simulink library "Driveline_Axle2_A1_A2_A1Diff_A2Diff"  (R2025a)
settings: Solver=VariableStepAuto  StartTime=0.0  StopTime=10.0  RelTol=1e-3
undefined symbols (not defined in the file): ShaftA1, ShaftA2
libraries: Driveshaft_Assembly x4, Differential_Systems x2, fl_lib x2, sdl_lib x2
Description:
  | Component of Simscape Vehicle Templates Library
  | 
  | Copyright 2018-2025 The MathWorks, Inc.
settings Model: Creator=smiller  LastModifiedBy=smiller
settings SolverCC: AlgebraicLoopSolver=TrustRegion
settings DataIOCC: ReturnWorkspaceOutputs=off
settings OptimizationCC: ReuseModelBlockBuffer=off
settings DebuggingCC: UnconnectedInputMsg=warning  UnconnectedOutputMsg=warning  UnconnectedLineMsg=warning  ArithmeticOperatorsInVariantConditions=warning
settings ModelReferenceCC: EnableRefExpFcnMdlSchedulingChecks=on
settings SFSimCC: CustomCodeUndefinedFunction=UseInterfaceOnly
settings RTWCC: GPUComputeCapability=3.5  DLArmComputeVersion=19.05

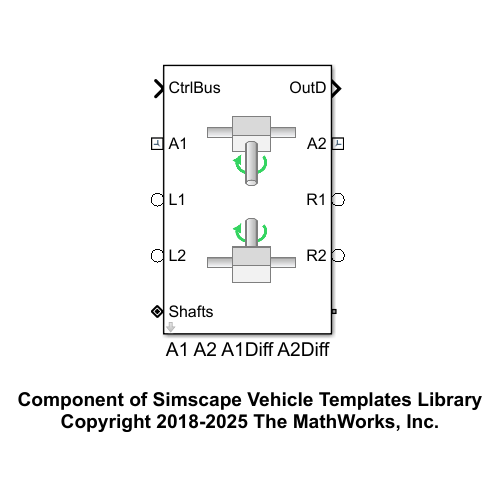
[thumbnail: Simulink's stored preview of the top-level diagram]
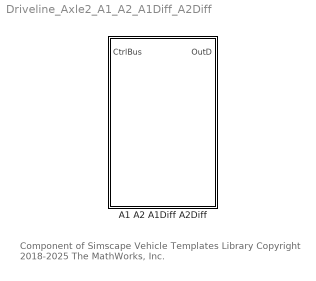
== system Driveline_Axle2_A1_A2_A1Diff_A2Diff ==
  note: Component of Simscape Vehicle Templates Library
      | Copyright 2018-2025 The MathWorks, Inc.
  A1 A2 A1Diff A2Diff : Subsystem  Tag=PublishSubsystem  VariantControl=IndepFRDiffFDiffR  mask(Driveline, Two-Axle, Two Input Shaft){}
      mask help: Models two-axle drivelines with differentials on front and rear axles.
      mask Display: image('sm_car_vehicle_driveline_axle2_a1_a2_a1diff_a2diff_IMAGE.png');

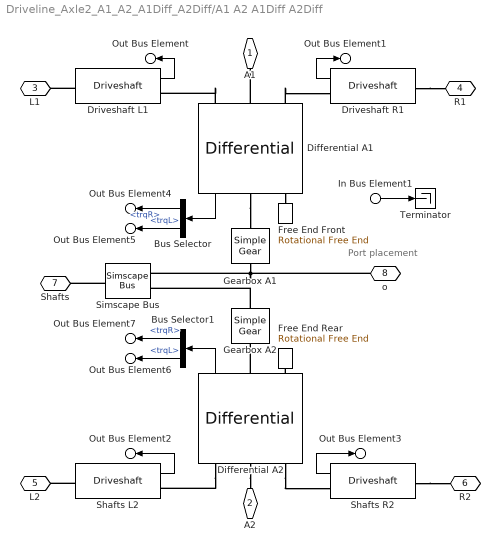
== system Driveline_Axle2_A1_A2_A1Diff_A2Diff/A1 A2 A1Diff A2Diff ==
  note: Port
      | placement
  In Bus Element1 : Inport  PortName=CtrlBus
  Bus Selector : BusSelector  OutputSignals=trqR,trqL
  Bus Selector1 : BusSelector  OutputSignals=trqR,trqL
  Differential A1 : Differential_Systems/Differential  VariantControl=Variant1  LabelModeActiveChoice=Gear1DShafts1D  Differential=Driveline.DifferentialA1  VariantLabel=Driveline.DifferentialA1.class.Value
      settings: AttributesFormatString=%<ActiveVariant>
  Differential A2 : Differential_Systems/Differential  VariantControl=Variant1  LabelModeActiveChoice=Gear1DShafts1D  Differential=Driveline.DifferentialA2  VariantLabel=Driveline.DifferentialA2.class.Value
      settings: AttributesFormatString=%<ActiveVariant>
  Driveshaft L1 : Driveshaft_Assembly/Driveshaft  VariantControl=Variant1  LabelModeActiveChoice=Shaft1D  popup_leftRight=Left  Driveshaft=Driveline.DriveshaftL1  VariantLabel=Driveline.DriveshaftL1.class.Value
      settings: AttributesFormatString=%<ActiveVariant>
  Driveshaft R1 : Driveshaft_Assembly/Driveshaft  VariantControl=Variant1  LabelModeActiveChoice=Shaft1D  popup_leftRight=Right  Driveshaft=Driveline.DriveshaftR1  VariantLabel=Driveline.DriveshaftR1.class.Value
      settings: AttributesFormatString=%<ActiveVariant>
  Free End Front : fl_lib/Mechanical/Rotational Elements/Rotational Free End  w_specify=off  w_priority=None  w=0 rad/s  w_nominal_specify=off  w_nominal_value=1  w_nominal_unit=rad/s
  Free End Rear : fl_lib/Mechanical/Rotational Elements/Rotational Free End  w_specify=off  w_priority=None  w=0 rad/s  w_nominal_specify=off  w_nominal_value=1  w_nominal_unit=rad/s
  Gearbox A1 : sdl_lib/Gears/Simple Gear  ratio=Driveline.GearboxA1.ratio.Value  rotation_direction=3-2*(1)  friction_model=1  T_noload=0.1 N*m  T_nom=5 N*m  efficiency_nom=0.8  efficiency=0.8  temperature_TLU=[280, 300, 320] K  load_TLU=[1, 5, 10] N*m  efficiency_TLU=[.95, .9, .85]  efficiency_TLU2=[.85, .8, .75; .95, .9, .85; .85, .8, .7]  w_thr=0.01 rad/s  pwr_thr=0.001 W  enable_backlash=false  hardstop_model=simscape.enum.hardstop.smooth  backlash_distance=1e-3 mm  r_base=0.1 m  transition=1e-4 mm  backlash_stiffness=1e7 N/m  backlash_damping=1e6 N*s/m  coeff_rest=0  v_tol=0.001 m/s  f_tol=0 N  mu_visc=[0, 0] N*m/(rad/s)  thermal_mass=50 J/K  temperature_specify=off  temperature_priority=High  temperature=300 K  temperature_nominal_specify=off  temperature_nominal_value=1  temperature_nominal_unit=K  x_backlash_specify=off  x_backlash_priority=None  x_backlash=0 mm  x_backlash_nominal_specify=off  x_backlash_nominal_value=1  x_backlash_nominal_unit=mm  f_hardstop_specify=off  f_hardstop_priority=None  f_hardstop=0 N  f_hardstop_nominal_specify=off  f_hardstop_nominal_value=1  f_hardstop_nominal_unit=N  v_backlash_specify=off  v_backlash_priority=None  v_backlash=0 m/s  v_backlash_nominal_specify=off  v_backlash_nominal_value=1  v_backlash_nominal_unit=m/s
  Gearbox A2 : sdl_lib/Gears/Simple Gear  ratio=Driveline.GearboxA2.ratio.Value  rotation_direction=3-2*(1)  friction_model=1  T_noload=0.1 N*m  T_nom=5 N*m  efficiency_nom=0.8  efficiency=0.8  temperature_TLU=[280, 300, 320] K  load_TLU=[1, 5, 10] N*m  efficiency_TLU=[.95, .9, .85]  efficiency_TLU2=[.85, .8, .75; .95, .9, .85; .85, .8, .7]  w_thr=0.01 rad/s  pwr_thr=0.001 W  enable_backlash=false  hardstop_model=simscape.enum.hardstop.smooth  backlash_distance=1e-3 mm  r_base=0.1 m  transition=1e-4 mm  backlash_stiffness=1e7 N/m  backlash_damping=1e6 N*s/m  coeff_rest=0  v_tol=0.001 m/s  f_tol=0 N  mu_visc=[0, 0] N*m/(rad/s)  thermal_mass=50 J/K  temperature_specify=off  temperature_priority=High  temperature=300 K  temperature_nominal_specify=off  temperature_nominal_value=1  temperature_nominal_unit=K  x_backlash_specify=off  x_backlash_priority=None  x_backlash=0 mm  x_backlash_nominal_specify=off  x_backlash_nominal_value=1  x_backlash_nominal_unit=mm  f_hardstop_specify=off  f_hardstop_priority=None  f_hardstop=0 N  f_hardstop_nominal_specify=off  f_hardstop_nominal_value=1  f_hardstop_nominal_unit=N  v_backlash_specify=off  v_backlash_priority=None  v_backlash=0 m/s  v_backlash_nominal_specify=off  v_backlash_nominal_value=1  v_backlash_nominal_unit=m/s
  Shafts L2 : Driveshaft_Assembly/Driveshaft  VariantControl=Variant1  LabelModeActiveChoice=Shaft1D  popup_leftRight=Left  Driveshaft=Driveline.DriveshaftL2  VariantLabel=Driveline.DriveshaftL2.class.Value
      settings: AttributesFormatString=%<ActiveVariant>
  Shafts R2 : Driveshaft_Assembly/Driveshaft  VariantControl=Variant1  LabelModeActiveChoice=Shaft1D  popup_leftRight=Right  Driveshaft=Driveline.DriveshaftR2  VariantLabel=Driveline.DriveshaftR2.class.Value
      settings: AttributesFormatString=%<ActiveVariant>
  Simscape Bus : SimscapeBus  HierarchyStrings=ShaftA1;ShaftA2
  Terminator : Terminator
  A1 : PMIOPort  Side=Left
  A2 : PMIOPort  Port=2  Side=Right
  L1 : PMIOPort  Port=3  Side=Left
  R1 : PMIOPort  Port=4  Side=Right
  L2 : PMIOPort  Port=5  Side=Left
  R2 : PMIOPort  Port=6  Side=Right
  Shafts : PMIOPort  Port=7  Side=Left
  o : PMIOPort  Port=8  Side=Right
  Out Bus Element6 : Outport  VectorParamsAs1DForOutWhenUnconnected=off  PortName=OutD  Element=MDriveshaftL2
  Out Bus Element7 : Outport  VectorParamsAs1DForOutWhenUnconnected=off  PortName=OutD  Element=MDriveshaftR2
  Out Bus Element4 : Outport  VectorParamsAs1DForOutWhenUnconnected=off  PortName=OutD  Element=MDriveshaftR1
  Out Bus Element5 : Outport  VectorParamsAs1DForOutWhenUnconnected=off  PortName=OutD  Element=MDriveshaftL1
  Out Bus Element : Outport  VectorParamsAs1DForOutWhenUnconnected=off  PortName=OutD  Element=anDriveshaftL1
  Out Bus Element1 : Outport  VectorParamsAs1DForOutWhenUnconnected=off  PortName=OutD  Element=anDriveshaftR1
  Out Bus Element2 : Outport  VectorParamsAs1DForOutWhenUnconnected=off  PortName=OutD  Element=anDriveshaftL2
  Out Bus Element3 : Outport  VectorParamsAs1DForOutWhenUnconnected=off  PortName=OutD  Element=anDriveshaftR2
  wires:
  In Bus Element1/1 -> Terminator/1
  Bus Selector/2 -> Out Bus Element5/1  "<trqL>"
  Bus Selector/1 -> Out Bus Element4/1  "<trqR>"
  Differential A2/1 -> Bus Selector1/1
  Bus Selector1/2 -> Out Bus Element6/1  "<trqL>"
  Bus Selector1/1 -> Out Bus Element7/1  "<trqR>"
  Differential A1/1 -> Bus Selector/1
  Shafts R2/1 -> Out Bus Element3/1
  Shafts L2/1 -> Out Bus Element2/1
  Driveshaft L1/1 -> Out Bus Element/1
  Driveshaft R1/1 -> Out Bus Element1/1
  connections:
  Simscape Bus/RConn1 -- Shafts/RConn1
  Differential A2/RConn1 -- Gearbox A2/RConn1
  Differential A2/LConn1 -- Shafts L2/RConn1
  Differential A2/LConn3 -- Shafts R2/RConn1
  Shafts L2/LConn1 -- L2/RConn1
  Shafts R2/LConn1 -- R2/RConn1
  Differential A1/RConn1 -- Gearbox A1/RConn1
  Differential A2/LConn2 -- A2/RConn1
  Differential A1/LConn2 -- A1/RConn1
  Driveshaft L1/LConn1 -- L1/RConn1
  Driveshaft R1/LConn1 -- R1/RConn1
  Differential A1/LConn3 -- Driveshaft R1/RConn1
  Differential A1/LConn1 -- Driveshaft L1/RConn1
  Differential A1/RConn2 -- Free End Front/LConn1
  Differential A2/RConn2 -- Free End Rear/LConn1
  Gearbox A1/LConn1 -- o/RConn1 -- Simscape Bus/LConn1
  Gearbox A2/LConn1 -- Simscape Bus/LConn2
